simulink model "gm_FPGA_SMC"  (R2019b)
settings: Solver=FixedStepAuto  StartTime=0.0  StopTime=10.0  RelTol=1e-3
libraries: hdlmdlgenlib x5
settings Model: Creator=Anas  LastModifiedBy=Anas
settings OptimizationCC: BlockReduction=off  ConditionallyExecuteInputs=off  EnhancedBackFolding=on  PassReuseOutputArgsAs=Individual arguments  ZeroExternalMemoryAtStartup=off  ZeroInternalMemoryAtStartup=off  MaxStackSize=64  OptimizeBlockOrder=speed  DifferentSizesBufferReuse=on  OptimizationCustomize=off  EfficientTunableParamExpr=on
settings DebuggingCC: InheritedTsInSrcMsg=none  ParameterTunabilityLossMsg=error
settings HardwareCC: ProdBitPerPointer=32  ProdBitPerSizeT=32  ProdBitPerPtrDiffT=32  ProdLargestAtomicFloat=None  ProdIntDivRoundTo=Undefined  ProdEndianess=Unspecified  ProdWordSize=32  ProdHWDeviceType=ASIC/FPGA->ASIC/FPGA  TargetBitPerPointer=64  TargetBitPerSizeT=64  TargetBitPerPtrDiffT=64  TargetLongLongMode=on  TargetIntDivRoundTo=Zero  TargetEndianess=LittleEndian  TargetWordSize=64  TargetHWDeviceType=Custom Processor->MATLAB Host Computer  ProdEqTarget=off  HardwareBoardFeatureSet=SoCBlockset
settings SFSimCC: MATLABDynamicMemAlloc=off
settings RTWCC: SystemTargetFile=ert.tlc  HardwareBoard=Custom Hardware Board  TLCOptions="-aInlineSetEventsForThisBaseRateFcn=TLC_FALSE -aSuppressMultiTaskScheduler=TLC_FALSE  -aRateBasedStepFcn=0"  TemplateMakefile=ert_default_tmf  GenerateReport=on  IncludeHyperlinkInReport=on  LaunchReport=on  GenerateTraceInfo=on  GenerateTraceReport=on  GenerateTraceReportSl=on  GenerateTraceReportSf=on  GenerateTraceReportEml=on
settings CodeAppCC: ForceParamTrailComments=on  IgnoreCustomStorageClasses=off  OperatorAnnotations=on  SimulinkDataObjDesc=on  SFDataObjDesc=on  InsertBlockDesc=on

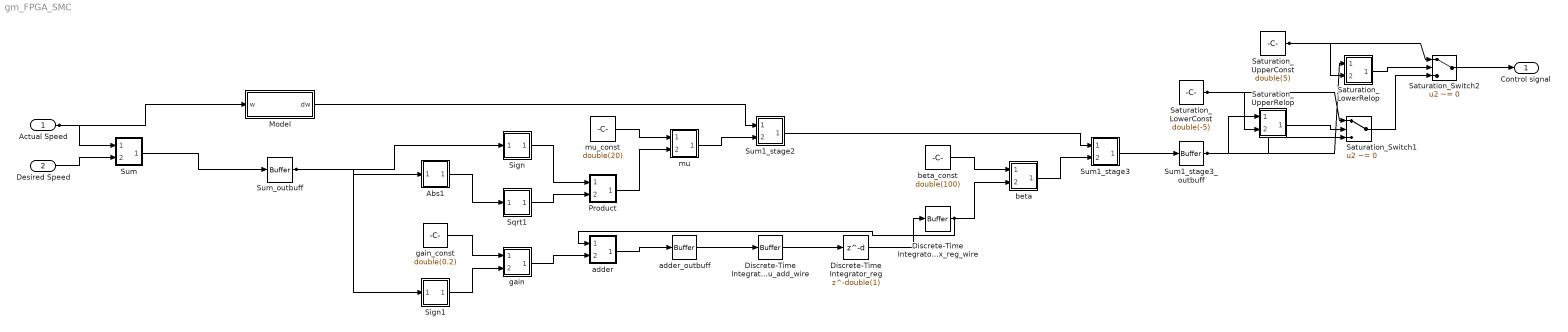
== system gm_FPGA_SMC ==
  Actual Speed : Inport  OutDataTypeStr=double  Unit=rad/sec  PortDimensions=1  SampleTime=0.2
  Desired Speed : Inport  Port=2  OutDataTypeStr=double  PortDimensions=1  SampleTime=0.2
  Abs1 : Subsystem
      mask Display: disp('NFP\nabs');
  Discrete-Time Integrator_reg : Delay  DelayLength=double(1)  InitialCondition=0  SampleTime=0.2
  Discrete-Time Integrator_u_add_wire : hdlmdlgenlib/Buffer
      settings: SourceProductName=Simulink  SourceProductBaseCode=SL
  Discrete-Time Integrator_x_reg_wire : hdlmdlgenlib/Buffer
      settings: SourceProductName=Simulink  SourceProductBaseCode=SL
  Model : Subsystem
  Product : Subsystem
      mask Display: disp('NFP\nmul');
  Saturation_LowerConst : Constant  Value=double(-5)  OutDataTypeStr=double  SampleTime=-1
  Saturation_LowerRelop : Subsystem
      mask Display: disp('NFP\nrelop');
  Saturation_Switch1 : Switch  Criteria=u2 ~= 0  Threshold=double(0)  OutDataTypeStr=double  SampleTime=0.2
  Saturation_Switch2 : Switch  Criteria=u2 ~= 0  Threshold=double(0)  OutDataTypeStr=double  SampleTime=0.2
  Saturation_UpperConst : Constant  Value=double(5)  OutDataTypeStr=double  SampleTime=-1
  Saturation_UpperRelop : Subsystem
      mask Display: disp('NFP\nrelop');
  Sign : Subsystem
      mask Display: disp('NFP\nsignum');
  Sign1 : Subsystem
      mask Display: disp('NFP\nsignum');
  Sqrt1 : Subsystem
      mask Display: disp('NFP\nsqrt');
  Sum : Subsystem
      mask Display: disp('NFP\nadd');
  Sum1_stage2 : Subsystem
      mask Display: disp('NFP\nadd');
  Sum1_stage3 : Subsystem
      mask Display: disp('NFP\nadd');
  Sum1_stage3_outbuff : hdlmdlgenlib/Buffer
      settings: SourceProductName=Simulink  SourceProductBaseCode=SL
  Sum_outbuff : hdlmdlgenlib/Buffer
      settings: SourceProductName=Simulink  SourceProductBaseCode=SL
  adder : Subsystem
      mask Display: disp('NFP\nadd');
  adder_outbuff : hdlmdlgenlib/Buffer
      settings: SourceProductName=Simulink  SourceProductBaseCode=SL
  beta : Subsystem
      mask Display: disp('NFP\nmul');
  beta_const : Constant  Value=double(100)  OutDataTypeStr=double  SampleTime=-1
  gain : Subsystem
      mask Display: disp('NFP\nmul');
  gain_const : Constant  Value=double(0.2)  OutDataTypeStr=double  SampleTime=-1
  mu : Subsystem
      mask Display: disp('NFP\nmul');
  mu_const : Constant  Value=double(20)  OutDataTypeStr=double  SampleTime=-1
  Control signal : Outport  VectorParamsAs1DForOutWhenUnconnected=off
  wires:
  Actual Speed/1 -> Sum/1(In1), Model/1(w)
  Desired Speed/1 -> Sum/2(In2)
  Discrete-Time Integrator_x_reg_wire/1 -> beta/2(In2), adder/1(In1)
  Model/1(dw) -> Sum1_stage2/1(In1)
  Saturation_Switch2/1 -> Control signal/1
  Sum_outbuff/1 -> Sign1/1(In1), Sign/1(In1), Abs1/1(In1)
  Sum1_stage3_outbuff/1 -> Saturation_LowerRelop/1(In1), Saturation_UpperRelop/1(In1), Saturation_Switch1/3
  adder_outbuff/1 -> Discrete-Time Integrator_u_add_wire/1
  Discrete-Time Integrator_u_add_wire/1 -> Discrete-Time Integrator_reg/1
  Discrete-Time Integrator_reg/1 -> Discrete-Time Integrator_x_reg_wire/1
  Saturation_LowerConst/1 -> Saturation_UpperRelop/2(In2), Saturation_Switch1/1
  Saturation_UpperConst/1 -> Saturation_LowerRelop/2(In2), Saturation_Switch2/1
  Saturation_Switch1/1 -> Saturation_Switch2/3
  gain_const/1 -> gain/1(In1)
  beta_const/1 -> beta/1(In1)
  mu_const/1 -> mu/1(In1)
  adder/1(Out1) -> adder_outbuff/1
  Abs1/1(Out1) -> Sqrt1/1(In1)
  Product/1(Out1) -> mu/2(In2)
  Saturation_UpperRelop/1(Out1) -> Saturation_Switch1/2
  Saturation_LowerRelop/1(Out1) -> Saturation_Switch2/2
  Sign/1(Out1) -> Product/1(In1)
  Sign1/1(Out1) -> gain/2(In2)
  Sqrt1/1(Out1) -> Product/2(In2)
  Sum/1(Out1) -> Sum_outbuff/1
  Sum1_stage2/1(Out1) -> Sum1_stage3/1(In1)
  Sum1_stage3/1(Out1) -> Sum1_stage3_outbuff/1
  gain/1(Out1) -> adder/2(In2)
  beta/1(Out1) -> Sum1_stage3/2(In2)
  mu/1(Out1) -> Sum1_stage2/2(In2)

== system gm_FPGA_SMC/Abs1 ==
  In1 : Inport
  Abs1 : Abs  SampleTime=0.2  OutDataTypeStr=double
  Out1 : Outport
  wires:
  In1/1 -> Abs1/1
  Abs1/1 -> Out1/1

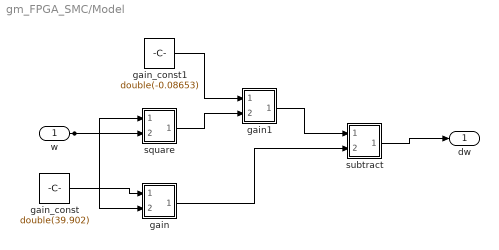
== system gm_FPGA_SMC/Model ==
  w : Inport  OutDataTypeStr=double  PortDimensions=1  SampleTime=0.2
  gain : Subsystem
      mask Display: disp('NFP\nmul');
  gain1 : Subsystem
      mask Display: disp('NFP\nmul');
  gain_const : Constant  Value=double(39.902)  OutDataTypeStr=double  SampleTime=-1
  gain_const1 : Constant  Value=double(-0.08653)  OutDataTypeStr=double  SampleTime=-1
  square : Subsystem
      mask Display: disp('NFP\nmul');
  subtract : Subsystem
      mask Display: disp('NFP\nadd');
  dw : Outport  VectorParamsAs1DForOutWhenUnconnected=off
  wires:
  w/1 -> gain/2(In2), square/2(In2), square/1(In1)
  gain_const/1 -> gain/1(In1)
  gain_const1/1 -> gain1/1(In1)
  subtract/1(Out1) -> dw/1
  square/1(Out1) -> gain1/2(In2)
  gain/1(Out1) -> subtract/2(In2)
  gain1/1(Out1) -> subtract/1(In1)

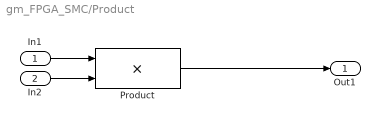
== system gm_FPGA_SMC/Product ==
  In1 : Inport
  In2 : Inport  Port=2
  Product : Product  Inputs=**  OutDataTypeStr=double  SampleTime=0.2
  Out1 : Outport
  wires:
  In1/1 -> Product/1
  In2/1 -> Product/2
  Product/1 -> Out1/1

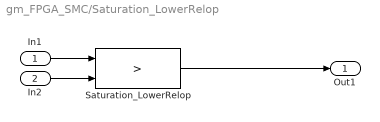
== system gm_FPGA_SMC/Saturation_LowerRelop ==
  In1 : Inport
  In2 : Inport  Port=2
  Saturation_LowerRelop : RelationalOperator  Operator=>  OutDataTypeStr=boolean  SampleTime=0.2  RndMeth=Nearest
  Out1 : Outport
  wires:
  In1/1 -> Saturation_LowerRelop/1
  In2/1 -> Saturation_LowerRelop/2
  Saturation_LowerRelop/1 -> Out1/1

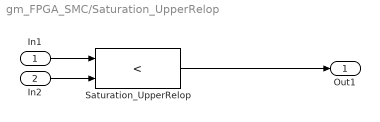
== system gm_FPGA_SMC/Saturation_UpperRelop ==
  In1 : Inport
  In2 : Inport  Port=2
  Saturation_UpperRelop : RelationalOperator  Operator=<  OutDataTypeStr=boolean  SampleTime=0.2  RndMeth=Nearest
  Out1 : Outport
  wires:
  In1/1 -> Saturation_UpperRelop/1
  In2/1 -> Saturation_UpperRelop/2
  Saturation_UpperRelop/1 -> Out1/1

== system gm_FPGA_SMC/Sign ==
  In1 : Inport
  Sign : Signum  SampleTime=0.2
  Out1 : Outport
  wires:
  In1/1 -> Sign/1
  Sign/1 -> Out1/1

== system gm_FPGA_SMC/Sign1 ==
  In1 : Inport
  Sign1 : Signum  SampleTime=0.2
  Out1 : Outport
  wires:
  In1/1 -> Sign1/1
  Sign1/1 -> Out1/1

== system gm_FPGA_SMC/Sqrt1 ==
  In1 : Inport
  Sqrt1 : Sqrt  SampleTime=0.2  IntermediateResultsDataTypeStr=double  SaturateOnIntegerOverflow=on
  Out1 : Outport
  wires:
  In1/1 -> Sqrt1/1
  Sqrt1/1 -> Out1/1

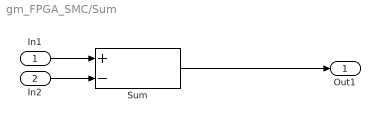
== system gm_FPGA_SMC/Sum ==
  In1 : Inport
  In2 : Inport  Port=2
  Sum : Sum  Inputs=+-  OutDataTypeStr=double  SampleTime=0.2  SaturateOnIntegerOverflow=on  InputSameDT=on
  Out1 : Outport
  wires:
  In1/1 -> Sum/1
  In2/1 -> Sum/2
  Sum/1 -> Out1/1

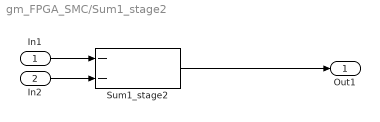
== system gm_FPGA_SMC/Sum1_stage2 ==
  In1 : Inport
  In2 : Inport  Port=2
  Sum1_stage2 : Sum  Inputs=--  OutDataTypeStr=double  SampleTime=0.2  SaturateOnIntegerOverflow=on  InputSameDT=on
  Out1 : Outport
  wires:
  In1/1 -> Sum1_stage2/1
  In2/1 -> Sum1_stage2/2
  Sum1_stage2/1 -> Out1/1

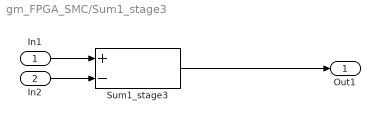
== system gm_FPGA_SMC/Sum1_stage3 ==
  In1 : Inport
  In2 : Inport  Port=2
  Sum1_stage3 : Sum  Inputs=+-  OutDataTypeStr=double  SampleTime=0.2  SaturateOnIntegerOverflow=on  InputSameDT=on
  Out1 : Outport
  wires:
  In1/1 -> Sum1_stage3/1
  In2/1 -> Sum1_stage3/2
  Sum1_stage3/1 -> Out1/1

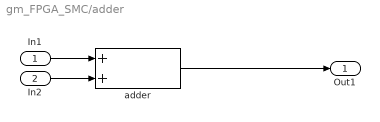
== system gm_FPGA_SMC/adder ==
  In1 : Inport
  In2 : Inport  Port=2
  adder : Sum  OutDataTypeStr=double  SampleTime=0.2  SaturateOnIntegerOverflow=on  InputSameDT=on
  Out1 : Outport
  wires:
  In1/1 -> adder/1
  In2/1 -> adder/2
  adder/1 -> Out1/1

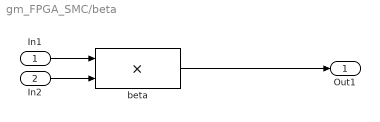
== system gm_FPGA_SMC/beta ==
  In1 : Inport
  In2 : Inport  Port=2
  beta : Product  Inputs=**  OutDataTypeStr=double  SampleTime=0.2
  Out1 : Outport
  wires:
  In1/1 -> beta/1
  In2/1 -> beta/2
  beta/1 -> Out1/1

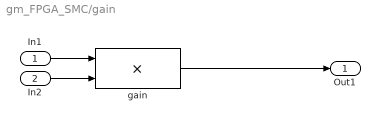
== system gm_FPGA_SMC/gain ==
  In1 : Inport
  In2 : Inport  Port=2
  gain : Product  Inputs=**  OutDataTypeStr=double  SampleTime=0.2
  Out1 : Outport
  wires:
  In1/1 -> gain/1
  In2/1 -> gain/2
  gain/1 -> Out1/1

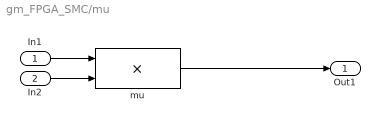
== system gm_FPGA_SMC/mu ==
  In1 : Inport
  In2 : Inport  Port=2
  mu : Product  Inputs=**  OutDataTypeStr=double  SampleTime=0.2
  Out1 : Outport
  wires:
  In1/1 -> mu/1
  In2/1 -> mu/2
  mu/1 -> Out1/1

== system gm_FPGA_SMC/Model/gain ==
  In1 : Inport
  In2 : Inport  Port=2
  gain : Product  Inputs=**  OutDataTypeStr=double  SampleTime=0.2
  Out1 : Outport
  wires:
  In1/1 -> gain/1
  In2/1 -> gain/2
  gain/1 -> Out1/1

== system gm_FPGA_SMC/Model/gain1 ==
  In1 : Inport
  In2 : Inport  Port=2
  gain1 : Product  Inputs=**  OutDataTypeStr=double  SampleTime=0.2
  Out1 : Outport
  wires:
  In1/1 -> gain1/1
  In2/1 -> gain1/2
  gain1/1 -> Out1/1

== system gm_FPGA_SMC/Model/square ==
  In1 : Inport
  In2 : Inport  Port=2
  square : Product  Inputs=**  OutDataTypeStr=double  SampleTime=0.2
  Out1 : Outport
  wires:
  In1/1 -> square/1
  In2/1 -> square/2
  square/1 -> Out1/1

== system gm_FPGA_SMC/Model/subtract ==
  In1 : Inport
  In2 : Inport  Port=2
  subtract : Sum  Inputs=+-  OutDataTypeStr=double  SampleTime=0.2  SaturateOnIntegerOverflow=on  InputSameDT=on
  Out1 : Outport
  wires:
  In1/1 -> subtract/1
  In2/1 -> subtract/2
  subtract/1 -> Out1/1
